simulink model "Theta2model"  (R2020a)
settings: Solver=VariableStepAuto  StartTime=0.0  StopTime=10.0  RelTol=1e-3
settings Model: Creator=marce  LastModifiedBy=marce

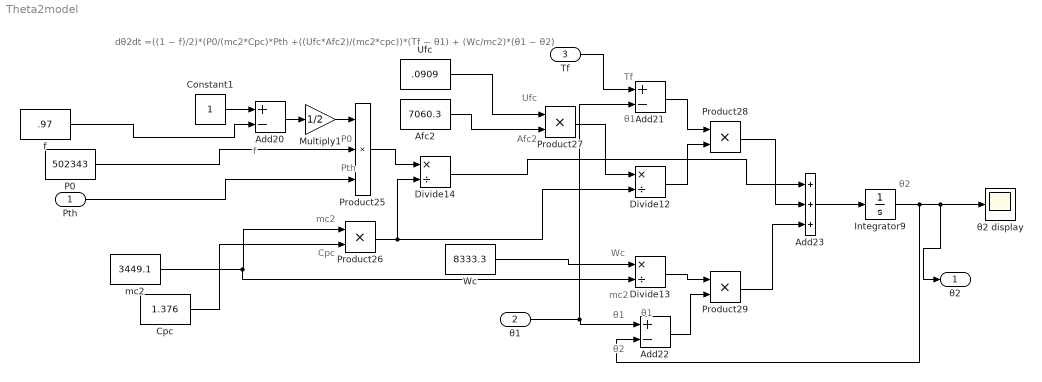
== system Theta2model ==
  note: Afc2
  note: Wc
  note: f
  note: Ufc
  note: mc2
  note: mc2
  note: θ1
  note: Cpc
  note: θ2
  note: θ1
  note: Tf
  note: P0
  note: θ1
  note: Pth
  note: θ2
  note: dθ2dt =((1 − f)/2)*(P0/(mc2*Cpc)*Pth +((Ufc*Afc2)/(mc2*cpc))*(Tf − θ1) + (Wc/mc2)*(θ1 − θ2)
  Pth : Inport
  θ1 : Inport  Port=2
  Tf : Inport  Port=3
  Add20 : Sum  Inputs=+-
  Add21 : Sum  Inputs=+-
  Add22 : Sum  Inputs=+-
  Add23 : Sum  Inputs=+++
  Afc2 : Constant  Value=7060.3
  Constant1 : Constant
  Cpc : Constant  Value=1.376
  Divide12 : Product  Inputs=*/
  Divide13 : Product  Inputs=*/
  Divide14 : Product  Inputs=*/
  Integrator9 : Integrator
  Multiply1 : Gain  Gain=1/2
  P0 : Constant  Value=502343
  Product25 : Product  Inputs=3
  Product{26..29} (4 alike) : Product
  Ufc : Constant  Value=.0909
  Wc : Constant  Value=8333.3
  f : Constant  Value=.97
  mc2 : Constant  Value=3449.1
  θ2 display : Scope
  θ2 : Outport
  wires:
  Product26/1 -> Divide12/2, Divide14/2
  Add23/1 -> Integrator9/1
  Add20/1 -> Multiply1/1
  Add22/1 -> Product29/2
  Divide12/1 -> Product28/2
  Multiply1/1 -> Product25/1
  Product28/1 -> Add23/2
  Product29/1 -> Add23/3
  Product25/1 -> Divide14/1
  Divide13/1 -> Product29/1
  Constant1/1 -> Add20/1
  Add21/1 -> Product28/1
  Integrator9/1 -> Add22/2, θ2/1, θ2 display/1
  Product27/1 -> Divide12/1
  Divide14/1 -> Add23/1
  f/1 -> Add20/2
  P0/1 -> Product25/2
  Pth/1 -> Product25/3
  mc2/1 -> Divide13/2, Product26/1
  Cpc/1 -> Product26/2
  Wc/1 -> Divide13/1
  θ1/1 -> Add21/2, Add22/1
  Ufc/1 -> Product27/1
  Afc2/1 -> Product27/2
  Tf/1 -> Add21/1
